simulink model "doc_gaussiantrig"  (R2014a)
settings: Solver=FixedStepDiscrete  SolverMode=SingleTasking  StartTime=0.0  StopTime=10  RelTol=1e-3
libraries: commnoisgen2 x2, dspsrcs4 x1
settings Model: Creator=The MathWorks Inc.
settings DataIOCC: SignalLoggingSaveFormat=ModelDataLogs
settings OptimizationCC: ExpressionDepthLimit=2147483647  InitFltsAndDblsToZero=on  EfficientMapNaN2IntZero=off
settings DebuggingCC: SaveWithParameterizedLinksMsg=none  UnderspecifiedInitializationDetection=Classic  SignalResolutionControl=TryResolveAllWithWarning  MultiTaskDSMMsg=warning  MultiTaskCondExecSysMsg=none  FcnCallInpInsideContextMsg=UseLocalSettings  StateNameClashWarn=warning  StrictBusMsg=None
settings RTWCC: IncludeERTFirstTime=on
settings GRTTargetCC: TargetFcnLib=ansi_tfl_tmw.mat  CombineOutputUpdateFcns=off  GRTInterface=on

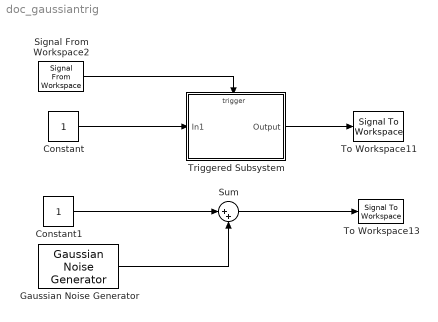
== system doc_gaussiantrig ==
  Constant : Constant  VectorParams1D=off  SampleTime=1
  Constant1 : Constant  VectorParams1D=off  SampleTime=1
  Gaussian Noise Generator : commnoisgen2/Gaussian Noise Generator  m=0  d=1  s=41  Ts=1  frameBased=on  sampPerFrame=1  orient=off  outDataType=double
  Signal From Workspace2 : dspsrcs4/Signal From Workspace  X=[0 1]  Ts=1  nsamps=1  OutputAfterFinalValue=Cyclic repetition  ignoreOrWarnInputAndFrameLengths=off
  Sum : Sum  Inputs=|++
  To Workspace11 : SignalToWorkspace  VariableName=trig_out
  To Workspace13 : SignalToWorkspace  VariableName=sim_out
  Triggered Subsystem : Subsystem  TreatAsAtomicUnit=on
  wires:
  Signal From Workspace2/1 -> Triggered Subsystem/Trigger
  Constant/1 -> Triggered Subsystem/1(In1)
  Triggered Subsystem/1(Output) -> To Workspace11/1
  Constant1/1 -> Sum/1
  Sum/1 -> To Workspace13/1
  Gaussian Noise Generator/1 -> Sum/2

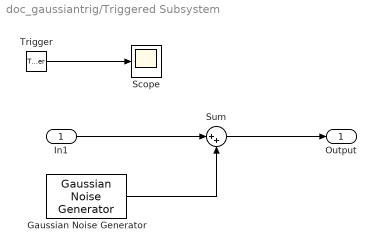
== system doc_gaussiantrig/Triggered Subsystem ==
  In1 : Inport
  Trigger : TriggerPort  ShowOutputPort=on
  Gaussian Noise Generator : commnoisgen2/Gaussian Noise Generator  m=0  d=1  s=41  Ts=-1  frameBased=on  sampPerFrame=1  orient=off  outDataType=double
  Scope : Scope
  Sum : Sum  Inputs=|++
  Output : Outport
  wires:
  In1/1 -> Sum/1
  Trigger/1 -> Scope/1
  Gaussian Noise Generator/1 -> Sum/2
  Sum/1 -> Output/1
